simulink model "CAVE_MachE_dSPACE_250912"  (R2024a)
settings: configuration reference "ConfigSetDesktopFixedStep" (kept outside this file)
PreLoadFcn:
  | VSS_BICYCLE=Simulink.Variant('Dual=0');
  | VSS_DUAL=Simulink.Variant('Dual=1');
  | Dual=1;
  | load('DriveCycle2.mat')
PostLoadFcn:
  | if any(exist('dsrtsu_mdlpostloadfcn', 'file') ~= 0), dsrtsu_mdlpostloadfcn('Execute', bdroot); end
InitFcn:
  | , if any(exist('rtifpga_mdlclblib', 'file') ~= 0), rtifpga_mdlclblib('Init', bdroot); end,
  | , if any(exist('dsmpb_private', 'file') ~= 0), dsmpb_private('dsmpb_mdlclblib', 'Init', bdroot); end,
  | load('DriveCycle2.mat')
model workspace (MAT data in the model file):
  Gas = 0.383333333333
values from neighbouring files (symbols this model uses):
  CoastDown =     [Run_Simulink.mat]
  limitedMCT =     [Run_Simulink.mat]
  MCT =     [Run_Simulink.mat]
  pMCT =     [Run_Simulink.mat]
  RealSimPara =     [Run_Simulink.mat]
  Ref_speed = [13 13.007895099 13.015778396 13.023649891 13.031509584 13.039357475 13.047193564 13.055017851 13.062830336 13.070631019 13.0784199 13.086196979 ... (2669 elements, 2669x1)]    [Ref_speed_and_time.mat]
  Ref_time = [0 0.01 0.02 0.03 0.04 0.05 0.06 0.07 0.08 0.09 0.1 0.11 ... (2669 elements, 2669x1)]    [Ref_speed_and_time.mat]
  US06 =     [Run_Simulink.mat]
undefined symbols (not defined in the file or in its folder): AccelCmd, ActTqLF_Nm_, ActTqLR_Nm_, ActTqRF_Nm_, ActTqRR_Nm_, BattChargeLimitMaxPwr, BattChargeLimitSocBpts, BattChargeLimitTbl, BattChrgCapcty, BattDischargeLimitSocBpts, BattDischargeLimitTbl, BattDischargeMaxPwr, BattNumCellsParallel, BattNumCellsSeries, BattOpenVoltCapBpts, BattOpenVoltTbl, BattResistSocBpts, BattResistTbl, BattResistTempBpts, BrakeMaxPrs, BrakeMaxTrq, ChassisDistCg2FrontAxle, ChassisDistCg2RearAxle, ChassisVehMass, CltchCmd, DecelCmd, DiffRatio, DiscIntNeverNeededParam, EnvGravCnst, EnvPrs, EnvTemp, FuelSpecificGrav, GearCmd, h, InitStates, lgSw, MtrEffSpdBpts, MtrEffTbl, MtrEffTrqBpts, MtrPwrMax, MtrTrqMax, SteeringCmd, SupvsryCtrlRegenBrkCutOffTbl, SupvsryCtrlRegenSpdBpts, TestScnrioCycleNum, VEH
libraries: VSIGenLib x122, simulink x112, etargetslib x75, dsmpblib x55, vehdynlibtire x24, CarMaker4SL x20, autolibshared x19, vehdynlibsuspension x14, vehdynlibtirecommon x14, autolibutils x10, VsrLibWheel x8, autolibpowerinfoutils x6
(part 1 of 31)
PreSaveFcn:
  | , if any(exist('dsmpb_private', 'file') ~= 0), dsmpb_private('dsmpb_mdlclblib', 'PreSave', bdroot); end,
CloseFcn:
  | , if any(exist('dsmpb_private', 'file') ~= 0), dsmpb_private('dsmpb_mdlclblib', 'Close', bdroot); end,
settings Model: DataDictionary=DdPassengerEv.sldd  DSMPB_ID_DATA={'18088',struct('BlockId','f88c42c2-e70e-4436-bd85-ff34452e836e','SignalIds',{{'1df572a0-f117-4729-9091-2c1a0a26ec90','0824b86c-995c-4624-95de-4f5a118cf0f7','1af539eb-325a-4e38-9107-84d6b0267392','ebb0fa34-559f-4fe0-b409-8a817ae8753c','d7145080-d35d-4c02-8c9e-cf76ffb14dc2','5075bfde-4142-4aeb-b309-025b37120541','abbab0bd-1456-4252-a37b-ee5f55ea0579','b5d617b8-bb24-4539-9145-e591a0a295f8','7df03788-1936-4801-98c0-dd7f6dfcacba','19949bfb-f246-4995-90e8-29a3751a0fa7','9454b59a-aedd-4270-89a6-1cca43305823','37cf720c-23c2-4b6d-8589-7b035c806643','98db9f76-eafd-4d54-90d2-d997d73b87d4','ff589fc8-5b21-4798-a75e-d26fc35c1fa1','e61b2882-e27e-4f06-b730-5e5281621b34','6605e0e6-8bf3-4a45-a0b0-4b9c1cf463f3','0d0f5161-daad-47a1-bb1d-ec2adbc183ca','48ba6675-0966-4a1c-b127-4f76dca3de94','3c897f11-b2eb-4eb8-b88f-7b7e913c6e41','378f468e-364f-43c5-91f9-fc8ddef6aca6','9c7f20ac-956d-4c19-bdea-31a2a3930ea2','bc252920-9c7c-4b91-a017-ee1d69e3f03c','a5e7a104-8664-4690-a58a-7cbf05737866','fe1cfa34-9b23-4225-85e3-0403f07d36e7','ab40d80a-815e-4994-aacd-e42d283f5b3a','2a4143b2-c438-4d42-997d-0587141eb8f0','2686c37a-8724-40b3-99fb-f8873ba286b8','3707aa1b-88c1-4f14-8f25-f346aa75c252','7413af4b-f834-4020-ad34-3dd98c546e0c','3445835b-9a90-4408-a32d-d76b66b0385b','23c9a144-1259-4fa3-9a16-4a32a7eadff9','5b4206b0-ea89-4111-86f7-7a4fd8c76b72','85c84ea6-72b6-4ccb-9199-727b305580c3','97bb0073-9d03-44a9-972d-49a0eb465678','8c3f0698-b0b6-4624-aa00-3a3096f7cc2f','c968922f-253e-433f-ad46-daf21e902962','21ad150a-19dc-415b-bc1b-b39528ec9221','a3572415-9467-4ff8-a492-c6c1b3cb1b64','700ac678-fb53-40b6-8e97-9eeffe7a1ca8','14ed5f8b-aa1d-402b-b493-5622a729893d','bdbcc0b3-c6a4-485e-8fbf-8c12a8df89e7','7a19cc2b-f06b-466f-ae52-fb8ac6fb0258','87deda6a-2251-4462-8ae0-a20845c776d4','41874d9b-304a-4265-a3a1-69d5c58383ea'}}),'18719',struct('BlockId','79daabbd-4df4-4017-ba65-d977f7e6cd2f','SignalIds',{{'63c99320-3a8a-469e-8a50-5c577229603f'}}),'18720',struct('BlockId','9f21d727-31d5-41b9-aed1-27a40d8edf8b','SignalIds',{{'abab19c9-0d91-46eb-acba-2a4710e305d8','b04a351a-0162-4e76-85ba-be44ac2701ab','ecceff37-eed3-4b02-b10b-52fe944a17cd'}}),'18721',struct('BlockId','5513e588-accc-447f-8233-209349c29c53','SignalIds',{{'cf7c35a9-6bda-4f5f-bfb5-f51ad44c376b'}}),'18722',struct('BlockId','a427ee23-ff95-4a9c-807f-ad2b61c33ee4','SignalIds',{{'b3e368f1-9670-4dd7-aa42-1fcccca64ddf'}}),'18723',struct('BlockId','53805a71-03ad-4b45-a2ab-66e4ec3700d0','SignalIds',{{'0801da20-d997-46db-8512-e37e1180e77c','d193450d-1a5a-4c8d-a2ac-d5fd306fefe3'}}),'18724',struct('BlockId','4d4909f9-4869-4ae2-8541-060fc5e29366','SignalIds',{{'0588d1ac-5d02-4ce0-9f56-5f4e572c1088','c0609b3e-104e-46bb-beb6-dc1d54d218ce','a0011887-c3f0-4769-95be-c916ccb77447','feb7a80d-e7d1-407d-8b44-49f086fb9d8a'}}),'42147',struct('BlockId','7c85148e-c3d7-432d-b81b-e11d436fb266','SignalIds',{{'d5c1f3b5-a22d-40e2-9adf-73dd3a0fe431'}}),'42148',struct('BlockId','5510fdf1-431a-410f-bcea-f7e8f570e2d1','SignalIds',{{'9fce7f97-eda7-4f24-878f-1a643d43b49c'}}),'42149',struct('BlockId','de0e2a2d-bbe1-43d1-85ae-8561a379e07c','SignalIds',{{'e73be657-c71a-4fa8-ab30-d8cdb28be71d'}}),'42224',struct('BlockId','1b1b092f-214b-4a80-b11b-37b75121e53b','SignalIds',{{'856b8b64-1382-4ba0-b818-e91eea7074c9'}}),'42225',struct('BlockId','cfba7721-c5cf-410b-a196-c40269978734','SignalIds',{{'7065876d-b123-4337-8b23-cec9822ec3f7'}}),'42226',struct('BlockId','45b8b98e-f988-42ef-b616-7180bc819cf2','SignalIds',{{'f4c7852e-b78f-4b21-ba9d-e4df57cf05c4'}}),'42232',struct('BlockId','ac7ecc60-8396-40a4-bc17-9f0f3c0759ca','SignalIds',{{'16a26856-ef2a-4966-8200-82aa3fe7ddbf'}}),'42233',struct('BlockId','13dab684-98bf-43e1-8dcd-5e4b904e530a','SignalIds',{{'2a6f66f1-336d-4450-a338-914a295f0636'}}),'42234',struct('BlockId','c2584fdd-8801-464b-b08c-93b745502641','SignalIds',{{'839033fa-96d7-490f-a336-e4074cb0a3a6'}}),'42263',struct('BlockId','5f5bdefb-1809-46da-bb29-06e43cb74cea','SignalIds',{{'9ba80473-de3d-4829-93f9-e3e4218e61ce'}}),'42264',struct('BlockId','3cf8559d-9792-4b7d-b1e9-07d3e8c975ef','SignalIds',{{'f258ffe4-6a36-4981-abe6-f58a11cec6e4'}}),'42772',struct('BlockId','2d079b89-a5d3-43f5-b2da-b67c6c9ddea6','SignalIds',{{'ca22f614-f5f3-4878-a32c-0e537783a285'}}),'42780',struct('BlockId','22a06564-7b80-437f-9a37-5f0480de49c5','SignalIds',{{'d3558271-70a3-4a15-b412-afa96387f019','02a3409b-9f87-437b-bf3a-cc29eabe585b','4dd1ea73-b952-4f27-91e5-448f679ccffd','2dcb7769-2bf3-4424-ac78-eb5f6dd54b66','045c974e-8d31-4d1e-8c69-be2d2594e84a'}}),'42781',struct('BlockId','f3d872af-dc59-442b-a387-2481dd52f459','SignalIds',{{'4ee2bd44-e8da-4e09-8a2d-8bab973be353','ce2328cf-0071-41cb-90b6-53c9d261887b'}}),'42785',struct('BlockId','b01cfdfa-14c4-45c6-876e-4dfb9db42377','SignalIds',{{'34ca8be0-54ab-4d71-8eb9-bde2ffc0f913'}}),'43275',struct('BlockId','53e01b05-b313-4d43-a0e9-b839859eb710','SignalIds',{{'161239c6-78c1-4aea-a8cb-c03beb6ae8ef'}}),'43351',struct('BlockId','937f730a-1a1f-4f40-8fb6-8c70050ca6d4','SignalIds',{{'ee16bc58-de2e-41bd-bfff-f1a6b1cd3b37','b53a6535-30cb-49b2-9826-525fa2ec09db','6c8ffc13-c120-49b6-9460-32fb34ba5a42','39b2e722-7db4-4c66-a473-01b75ecb1f7e','6185bd49-892f-4e96-a0db-104c5534c4be'}}),'49495',struct('BlockId','35ff131a-9de8-4d32-b660-bb6fceef702f','SignalIds',{{'b3d83f02-eed5-45fe-aef0-78174e9f35bd'}}),'49496',struct('BlockId','bf00eff8-ae28-429c-ab8a-46a75e93ba18','SignalIds',{{'86a9df83-1438-4adb-98b7-232805926a36'}}),'49497',struct('BlockId','d54ce848-7528-4eb9-ae42-5423de96ecef','SignalIds',{{'e89a887d-f88e-44f1-b02b-282b9de2f1ab'}}),'49572',struct('BlockId','c08c591c-899c-44b3-88ca-9869f13035b2','SignalIds',{{'eb7d554f-c70c-43ca-87de-5673b1b09813'}}),'49573',struct('BlockId','9ed6cbeb-a118-471e-b0e5-7b29cbd80ac9','SignalIds',{{'e78b4934-46c3-41f5-baf1-b0c8a26c6d3b'}}),'49574',struct('BlockId','61fba3a3-d3ec-4ab0-be81-a8cb14a538ce','SignalIds',{{'aafde299-1c10-4ae2-865d-2eebd2e1d68a'}}),'49580',struct('BlockId','895e4f2c-adf9-4e1f-babd-51f59cfff5b5','SignalIds',{{'825a4d44-3ac8-4ffd-9f33-50dd2ede91f2'}}),'49581',struct('BlockId','65ead0f7-0652-4680-9e89-6e39b662d157','SignalIds',{{'833f3807-08e2-419e-8eac-d416545ff0e8'}}),'49582',struct('BlockId','ae266637-3823-4e51-9a5d-b81a88878ea4','SignalIds',{{'7abd4bb8-4f81-4261-991b-ba40c4239b3f'}}),'49611',struct('BlockId','77863ddb-e348-485a-81f5-f37c73594fca','SignalIds',{{'b85974cd-0117-43cc-9e24-4cf6f83a5038'}}),'49612',struct('BlockId','8a6bfe7e-fecd-4338-b064-35f762c57dd4','SignalIds',{{'028a9207-fccc-429b-a69c-4f023900ccb5'}}),'50148',struct('BlockId','d1cbcaa1-cb10-47dc-bb74-55eff0f5b43b','SignalIds',{{'203ceee9-7451-4837-a304-33672f7cb3bd'}}),'50156',struct('BlockId','7627d88c-f2e4-403d-80ba-43b5276eda68','SignalIds',{{'322b732d-d2d2-46e4-9338-f008ec14fc06','19c378a0-40df-4104-b400-16195277658b','129b4dde-e693-4553-ada1-0a9cf8694d1d','28bef0ec-e017-4484-a602-27bf02ddcdfb','d37ce16d-143d-4750-b239-1ca329bec6cc'}}),'50157',struct('BlockId','caace046-61cc-4e48-8b3d-a44e7bf76e0c','SignalIds',{{'2a1998fe-82ad-4e18-9452-adc54fc26a08','16216acf-8215-436c-93b3-ee24dac643a7'}}),'50161',struct('BlockId','87d87a7c-a686-43fe-9c61-68513704cc99','SignalIds',{{'b845dc9e-5d72-4a9d-93ac-413a3cfc992f'}}),'50651',struct('BlockId','00e0e527-d2ca-4571-801c-cfc2bc29d995','SignalIds',{{'b4404b90-9372-444b-968a-2bd31005b611'}}),'50727',struct('BlockId','25b59a2e-42b7-4e07-879c-15e188342b70','SignalIds',{{'e976513c-fd89-4869-a98f-324219a9d934','829bf17c-2f45-4024-9dab-76a03bee14cf','0e1b211c-e5c6-4562-ba57-cff21183358a','56f35125-16f5-4225-9f4e-e6e61c42686e','40167815-fad9-4050-b1e6-1da6841d0f65'}}),'53300',struct('BlockId','ae15802c-8b47-4761-960d-0ebe7bc28239','SignalIds',{{'650e13a2-8980-4a2b-ad4a-82bd33536a23'}}),'53322',struct('BlockId','ff36f65e-48c3-4e0a-8bc0-4b163bd9adbf','SignalIds',{{'5a20c0d4-68ad-414c-b231-cbf9ddd3e095'}}),'53323',struct('BlockId','ff546a49-594f-4f8a-affd-90d138806f61','SignalIds',{{'5fe60c73-3931-4298-88e1-7e5400488d1f','248c84a0-5741-40b6-9df8-c31abbb2257e','cca71626-162d-41c0-b616-b3a204f50bd7','6e7b0574-cba0-4ecc-ac4f-9c1d2acf4299'}}),'53324',struct('BlockId','a705fb28-535c-4f81-ad43-e460cea2d9bd','SignalIds',{{'398a40fd-c49e-4cdc-b573-2bb4186f6a80'}}),'53325',struct('BlockId','640f6546-7547-4622-bc5f-0a859f60736c','SignalIds',{{'f16056a3-5355-45cf-b9ed-57b3d5aab693'}}),'53330',struct('BlockId','93c276bb-de34-4a5c-95b3-f478e766cc9c','SignalIds',{{'c132201b-d036-47bb-91a2-a150e3b7ae13','ab601218-fa7c-4092-949e-1c1efb88023c'}}),'53343',struct('BlockId','8d0d14d0-22eb-49b1-810b-505b992714e9','SignalIds',{{'23156721-17dc-438a-8419-66eeaab95ef6','031c7289-7cec-4992-a9bf-cac5b5fae03e','ee32aa15-99a4-47b6-971a-419c12efa46a'}}),'53436',struct('BlockId','f41b78f3-d575-41ef-a146-3918605c1ef5','SignalIds',{{'e2c9672b-95ca-4046-bb0a-7aa2ea23f667'}}),'53439',struct('BlockId','d56f2d58-e632-40cf-b303-c9d86bf84e1a','SignalIds',{{'59ee7074-abb0-4813-a7c7-2ef1cc941406'}}),'53488',struct('BlockId','418072fe-6709-46db-9629-338ace776db3','SignalIds',{{'044486e3-c8e5-469a-9e14-4b7ebf45cbba','40dd4e22-2973-48dc-8d39-42c08d6738c4'}}),'53490',struct('BlockId','7526ad31-4259-4e92-8867-16b3b004889f','SignalIds',{{'fba7c128-fffd-4ae7-8d8c-de066c2017dd'}}),'53491',struct('BlockId','062ca957-a507-4bdc-8288-474fbe5dbd0f','SignalIds',{{'af7253ef-dad5-44d9-bc07-eac7de166a86','3be6fa1b-709c-42ac-b822-ca052c4e2367','f965bb3f-6162-4a13-806f-161423ed84b7'}}),'53492',struct('BlockId','fc9bee8e-3606-4482-8e61-57f769d8705e','SignalIds',{{'08427df5-b687-45d9-8b32-97283f4d5ce7'}}),'53509',struct('BlockId','bc68f02f-4d7c-4dde-a2d1-5019dce219ff','SignalIds',{{'21518aaf-593c-482f-a05c-e4a1b5e97c9f','b433a259-e771-4f81-a0d0-6fb158bd2e5d','6775e424-27e2-42c2-9fab-4841f171aca3','bf8792cd-664c-41ca-8c7b-827f476f84f2'}})}  RTICANMMDATA=struct('GeneralSetupData',struct('modelroot','C:\GitDev\Anye\cave_carla_dev\Vehicles\VehicleProjects\Bolt_EV\System','generalsettings',struct('filesettings',struct('destfolder',struct('Name','RTICANMM_FILES','Check',1),'buildfolder',struct('Name','.','Check',1),'AbsDestfolder',struct('Name','C:\GitDev\Anye\cave_carla_dev\Vehicles\VehicleProjects\Bolt_EV\System\RTICANMM_FILES'),'AbsBuildfolder',struct('Name','C:\GitDev\Anye\cave_carla_dev\Vehicles\VehicleProjects\Bolt_EV\System'))),'options',struct('addpaths',1,'rmpaths',1,'addtrcexclusion',true,'cannavigator',struct('checkmonitoring',0),'show_usrtrc',0,'use_usrtrc',0),'advanced',struct('options',ones(1,100)),'MPSetup',{{}},'RTI',struct('Type','DSRT','Ver','4.2p1','Date','11-Feb-2020'),'modelname','CAVE_MachE','block','CAVE_MachE'))  DSRTSU_INTERNAL_RTIFPGA=210  DSRTSU_INTERNAL_RTISTBM_VER=24.1  PauseTimes=45  Creator=9bt  LastModifiedBy=MSC_Lab
settings ConfigSetRef: SourceName=ConfigSetDesktopFixedStep

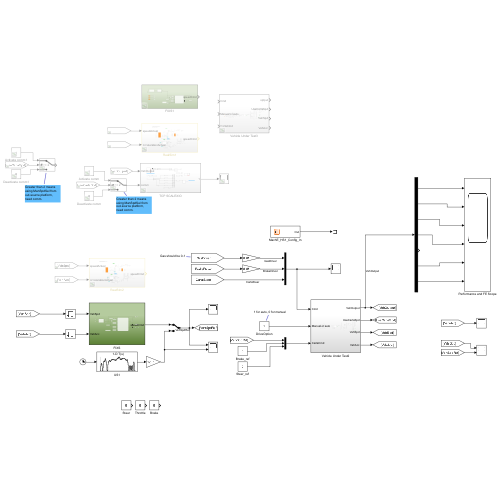
[thumbnail: Simulink's stored preview of the top-level diagram]
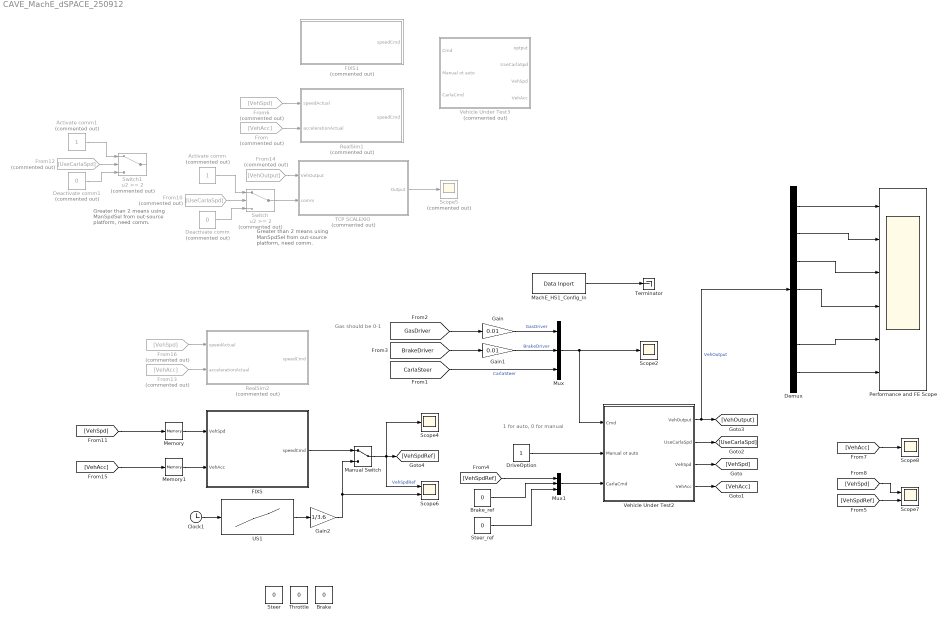
== system CAVE_MachE_dSPACE_250912 ==
  note: Greater than 2 means using ManSpdSel from out-source platform, need comm.
  note: 1 for auto, 0 for manual
  note: Gas should be 0-1
  note: Greater than 2 means using ManSpdSel from out-source platform, need comm.
  Activate comm : Constant  Commented=on
  Activate comm1 : Constant  Commented=on
  Brake : Constant  Value=0
  Brake_ref : Constant  Value=0
  Clock1 : Clock
  Deactivate comm : Constant  Commented=on  Value=0
  Deactivate comm1 : Constant  Commented=on  Value=0
  Demux : Demux  Outputs=7
  DriveOption : Constant
  FIXS : Subsystem
  FIXS1 : Subsystem  Commented=on
  From : From  Commented=on  GotoTag=VehAcc
  From10 : From  Commented=on  GotoTag=UseCarlaSpd
  From12 : From  Commented=on  GotoTag=UseCarlaSpd
  From13 : From  Commented=on  GotoTag=VehAcc
  From14 : From  Commented=on  GotoTag=VehOutput
  From16 : From  Commented=on  GotoTag=VehSpd
  From6 : From  Commented=on  GotoTag=VehSpd
  Gain : Gain  Gain=0.01
  Gain1 : Gain  Gain=0.01
  Gain2 : Gain  Gain=1/3.6
  MachE_HS1_Config_In : dsmpblib/Data Inport  Priority=10000
      settings: SourceProductName=dSPACE Model Interface Package for Simulink (MIPS)
  Manual Switch : ManualSwitch
  Memory : Memory
  Memory1 : Memory
  Mux : Mux  Inputs=3
  Mux1 : Mux  Inputs=3
  Performance and FE Scope : Scope  NumInputPorts=6
  RealSim1 : Subsystem  Commented=on
  RealSim2 : Subsystem  Commented=on
  Scope2 : Scope
  Scope4 : Scope
  Scope5 : Scope  Commented=on
  Scope6 : Scope  NumInputPorts=2
  Scope7 : Scope  NumInputPorts=2
  Scope8 : Scope
  Steer : Constant  Value=0
  Steer_ref : Constant  Value=0
  Switch : Switch  Commented=on  Threshold=2  SaturateOnIntegerOverflow=off  InputSameDT=off
  Switch1 : Switch  Commented=on  Threshold=2  SaturateOnIntegerOverflow=off  InputSameDT=off
  TCP SCALEXIO : Subsystem  Commented=on
  Terminator : Terminator
  Throttle : Constant  Value=0
  US1 : Lookup_n-D  NumberOfTableDimensions=1  BreakpointsForDimension1=US06.Time  Table=US06.Speed  InternalRulePriority=Speed  RndMeth=Simplest
  Vehicle Under Test2 : Subsystem
  Vehicle Under Test3 : Subsystem  Commented=on
  wires:
  Mux/1 -> Vehicle Under Test2/1(Cmd), Scope2/1
  DriveOption/1 -> Vehicle Under Test2/2(Manual ot auto)
  [GasDriver] -> Gain/1
  [BrakeDriver] -> Gain1/1
  MachE_HS1_Config_In/1 -> Terminator/1
  Gain/1 -> Mux/1  "GasDriver"
  Gain1/1 -> Mux/2  "BrakeDriver"
  Vehicle Under Test2/1(VehOutput) -> [VehOutput], Demux/1  "VehOutput"
  Switch/1 -> TCP SCALEXIO/2(comm)
  TCP SCALEXIO/1(Output) -> Scope5/1
  Deactivate comm/1 -> Switch/3
  Activate comm/1 -> Switch/1
  [CarlaSteer] -> Mux/3  "CarlaSteer"
  Manual Switch/1 -> Scope4/1, Scope6/1, [VehSpdRef]  "VehSpdRef"
  US1/1 -> Gain2/1
  From/1 -> RealSim1/2(accelerationActual)
  From6/1 -> RealSim1/1(speedActual)
  [VehSpdRef] -> Mux1/1
  Mux1/1 -> Vehicle Under Test2/3(CarlaCmd)
  Vehicle Under Test2/3(VehSpd) -> [VehSpd]
  Vehicle Under Test2/4(VehAcc) -> [VehAcc]
  Steer_ref/1 -> Mux1/3
  Brake_ref/1 -> Mux1/2
  Vehicle Under Test2/2(UseCarlaSpd) -> [UseCarlaSpd]
  Clock1/1 -> US1/1
  [VehSpdRef] -> Scope7/2
  Gain2/1 -> Scope6/2, Manual Switch/2
  Demux/1 -> Performance and FE Scope/1
  Demux/7 -> Performance and FE Scope/6
  Demux/6 -> Performance and FE Scope/5
  Demux/4 -> Performance and FE Scope/4
  Demux/3 -> Performance and FE Scope/3
  Demux/2 -> Performance and FE Scope/2
  [VehAcc] -> Scope8/1
  [VehSpd] -> Scope7/1
  From10/1 -> Switch/2
  [VehSpd] -> Memory/1
  FIXS/1(speedCmd) -> Manual Switch/1
  From12/1 -> Switch1/2
  Activate comm1/1 -> Switch1/1
  Deactivate comm1/1 -> Switch1/3
  From14/1 -> TCP SCALEXIO/1(VehOutput)
  [VehAcc] -> Memory1/1
  From16/1 -> RealSim2/1(speedActual)
  From13/1 -> RealSim2/2(accelerationActual)
  Memory/1 -> FIXS/1(VehSpd)
  Memory1/1 -> FIXS/2(VehAcc)

== system CAVE_MachE_dSPACE_250912/FIXS ==
  note: This flag will bypass all other logic and force the ramp down of HIL
  VehSpd : Inport
  VehAcc : Inport  Port=2
  Clock : Clock
  Constant : Constant  Value=RealSimPara.speedInit
  DistanceTravel (m) : Constant  Value=0
  Gain3 : Gain  Gain=3.6
  Manual Switch : ManualSwitch  CurrentSetting=0
  Manual Switch1 : ManualSwitch
  RampDownFlag : Constant  Value=0
  RampUpFlag : Constant  Value=0
  RealSim Core : Subsystem
  RealSimHILCycle : Stateflow chart  TreatAsAtomicUnit=on
  SimState : Constant  Value=10
  SimTime : Constant  Value=10
  Terminator{,1..4} (5 alike) : Terminator
  initialWaitTime : Constant  Value=0
  totalDistance (m) : Constant  Value=1000000
  totalTime (sec) : Constant  Value=10000
  speedCmd : Outport
  wires:
  RealSim Core/2(speedDesiredIn) -> Terminator/1
  RampDownFlag/1 -> RealSimHILCycle/9(RampDownFlag)
  totalDistance (m)/1 -> RealSimHILCycle/7(totalDistance)
  Manual Switch/1 -> RealSimHILCycle/3(SpeedIn)
  Gain3/1 -> Terminator1/1  "HIL_SpeedCmd_kph"
  totalTime (sec)/1 -> RealSimHILCycle/8(totalTime)
  RealSimHILCycle/1(CycleMode) -> Terminator3/1  "CycleMode"
  initialWaitTime/1 -> RealSimHILCycle/5(InitWaitTime)
  RealSimHILCycle/2(SpeedCmd) -> [HIL_SpeedCmd], Manual Switch1/2, Gain3/1
  Constant/1 -> Manual Switch/1, RealSimHILCycle/6(SpeedInit)
  Manual Switch1/1 -> speedCmd/1
  RealSim Core/3(speedCmd) -> Manual Switch1/1, Manual Switch/2
  RampUpFlag/1 -> RealSimHILCycle/10(RampUpFlag)
  VehSpd/1 -> RealSim Core/1(VehSpd)
  RealSim Core/1(VehDataBusIn) -> Terminator2/1
  RealSim Core/4(speedActual) -> Terminator4/1
  DistanceTravel (m)/1 -> RealSimHILCycle/4(DistanceTravel)
  SimState/1 -> RealSimHILCycle/2(SimState)
  Clock/1 -> RealSimHILCycle/1(SimTime)
  VehAcc/1 -> RealSim Core/2(VehAcc)

== system CAVE_MachE_dSPACE_250912/FIXS1 ==
  note: This flag will bypass all other logic and force the ramp down of HIL
  Constant : Constant  Value=RealSimPara.speedInit
  Gain3 : Gain  Gain=3.6
  Manual Switch : ManualSwitch  CurrentSetting=0
  Manual Switch1 : ManualSwitch  CurrentSetting=0
  RampDownFlag : Constant  Value=0
  RampUpFlag : Constant  Value=0
  Read CM Dict3 : CarMaker4SL/Read CM Dict  xname=Time  xsync=off  xstime=Continuous
  Read CM Dict7 : CarMaker4SL/Read CM Dict  xname=SC.State  xsync=off  xstime=Continuous
  Read CM Dict8 : CarMaker4SL/Read CM Dict  xname=Vhcl.Distance  xsync=off  xstime=Continuous
  RealSim Core : Subsystem
  RealSim Translate CM Signal to Bus as Feedback to SUMO/VISSIM : Subsystem
  RealSimHILCycle : Stateflow chart  TreatAsAtomicUnit=on
  Terminator : Terminator
  Terminator1 : Terminator
  Terminator3 : Terminator
  initialWaitTime : Constant  Value=10000
  totalDistance (m) : Constant  Value=1000000
  totalTime (sec) : Constant  Value=10000
  speedCmd : Outport
  wires:
  RealSim Translate CM Signal to Bus as Feedback to SUMO/VISSIM/1(VehDataBusOut) -> RealSim Core/1(VehDataBusOut)
  RealSim Core/2(speedDesiredIn) -> Terminator/1
  RealSim Core/1(VehDataBusIn) -> RealSim Translate CM Signal to Bus as Feedback to SUMO/VISSIM/1(VehDataBusIn)
  RealSim Translate CM Signal to Bus as Feedback to SUMO/VISSIM/2(CM_speed) -> RealSim Core/2(CM_speed)
  RampDownFlag/1 -> RealSimHILCycle/9(RampDownFlag)
  totalDistance (m)/1 -> RealSimHILCycle/7(totalDistance)
  Manual Switch/1 -> RealSimHILCycle/3(SpeedIn)
  Gain3/1 -> Terminator1/1  "HIL_SpeedCmd_kph"
  totalTime (sec)/1 -> RealSimHILCycle/8(totalTime)
  RealSimHILCycle/1(CycleMode) -> Terminator3/1  "CycleMode"
  initialWaitTime/1 -> RealSimHILCycle/5(InitWaitTime)
  RealSimHILCycle/2(SpeedCmd) -> [HIL_SpeedCmd], Manual Switch1/2, Gain3/1
  Constant/1 -> RealSimHILCycle/6(SpeedInit), Manual Switch/1
  [DistanceTravel] -> RealSimHILCycle/4(DistanceTravel)
  [SimState] -> RealSimHILCycle/2(SimState)
  [CM_Time] -> RealSimHILCycle/1(SimTime)
  Manual Switch1/1 -> speedCmd/1
  RealSim Core/3(speedCmd) -> Manual Switch/2, Manual Switch1/1
  Read CM Dict7/1 -> [SimState]  "SimCore_State"
  Read CM Dict8/1 -> [DistanceTravel]  "distanceTravel"
  Read CM Dict3/1 -> [CM_Time]  "CM_Time"
  RampUpFlag/1 -> RealSimHILCycle/10(RampUpFlag)
  RealSim Core/4(speedActual) -> RealSim Translate CM Signal to Bus as Feedback to SUMO/VISSIM/2(speedActual)

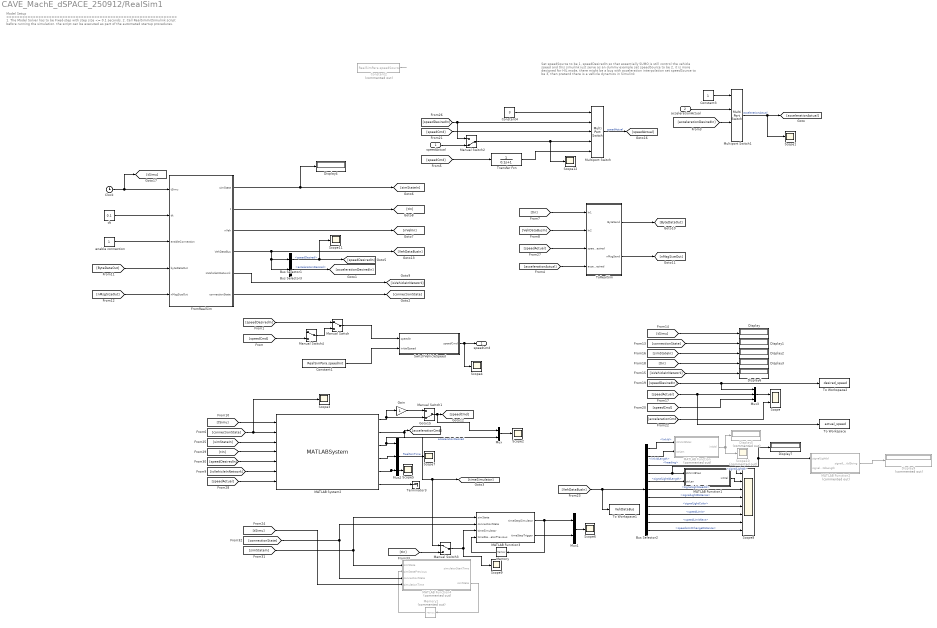
== system CAVE_MachE_dSPACE_250912/RealSim1 ==
  note: Set speedSource to be 1, speedDesiredIn so that essentially SUMO is still control the vehicle speed and this simulink just serve as an dummy example
      |
      | set speedSource to be 2, it is more designed for HIL mode, there might be a bug with acceleration interpolation
      |
      | set speedSource to be 3, then pretend there is a vehicle dynamics in Simulink
  note: Model Setup
      | ================================================================
      | 1. The Model Solver has to be Fixed-step with step size <= 0.1 seconds.
      | 2. Call RealSimInitSimulink script before running the simulation. the script can be executed as part of the automated startup procedures.
  speedActual : Inport
  accelerationActual : Inport  Port=2
  Bus Selector1 : BusSelector  OutputSignals=speedDesired
  Bus Selector2 : BusSelector  OutputSignals=linkId,linkIdLength,heading,signalLightId,signalLightIdLength,signalLightHeadId,signalLightDistance,signalLightColor,speedLimit,speedLimitNext,speedLimitChangeDistance
  Bus Selector3 : BusSelector  OutputSignals=accelerationDesired
  Clock : Clock
  Constant1 : Constant  Value=RealSimPara.speedInit
  Constant2 : Constant  Commented=on  Value=RealSimPara.speedSource
  Constant3 : Constant
  Constant4 : Constant  Value=3
  Display{,1..4,6..7} (7 alike) : Display
  Display5 : Display  Commented=on
  Display9 : Display  Commented=on
  FromRealSim : Subsystem
  Gain : Gain
  MATLAB Function : MATLAB Function  Commented=on  TreatAsAtomicUnit=on
  MATLAB Function1 : MATLAB Function  TreatAsAtomicUnit=on
  MATLAB Function2 : MATLAB Function  Commented=on  TreatAsAtomicUnit=on  SystemSampleTime=0.001
  MATLAB Function3 : MATLAB Function  TreatAsAtomicUnit=on
  MATLAB Function4 : MATLAB Function  Commented=on  TreatAsAtomicUnit=on
  MATLAB System2 : MATLABSystem  System=RealSimInterpSpeed  initialSpeed=RealSimPara.speedInit  speedLookAheadHorizon=RealSimPara.tLookahead  speedUpperBound=30  smoothWindow=RealSimPara.smoothWindow  SimulateUsing=Interpreted execution
      mask Type: RealSimInterpSpeed
      mask Display:
      | disp('RealSimInterpSpeed');
      | port_label('input',1,'simulationTime');
      | port_label('input',2,'connectionState');
      | port_label('input',3,'simState');
      | port_label('input',4,'timeReceive');
      | port_label('input',5,'speedReceive');
      | port_label('input',6,'isVehicleInNetwork');
      | port_label('input',7,'speedActual');
      | port_label('output',1,'speedLookAhead');
      | port_label('output',2,'accelerationDesired');
      | port_label('output',3,'timeSimulator');
      | port_label('output',4,'timeStepSimulator');
      | port_label('output',5,'timeStepTrigger');
      | port_label('output',6,'RealSimDelay');
  Manual Switch : ManualSwitch
  Manual Switch1 : ManualSwitch  CurrentSetting=0
  Manual Switch2 : ManualSwitch  CurrentSetting=0
  Manual Switch3 : ManualSwitch
  Manual Switch4 : ManualSwitch
  Memory : Memory
  Memory1 : Memory  Commented=on
  Multiport Switch : MultiPortSwitch  Inputs=4  SaturateOnIntegerOverflow=off  InputSameDT=off
  Multiport Switch1 : MultiPortSwitch  SaturateOnIntegerOverflow=off  InputSameDT=off
  Mux : Mux  Inputs=2
  Mux1 : Mux  Inputs=2
  Mux2 : Mux  Inputs=3
  Mux3 : Mux  Inputs=3
  Scope : Scope  NumInputPorts=2
  Scope{1..7,9,11..12} (10 alike) : Scope
  Scope10 : Scope  Commented=on
  Scope8 : Scope  NumInputPorts=8
  SwitchVehicleSpeed : Subsystem
  Terminator3 : Terminator
  To Workspace : ToWorkspace  VariableName=actual_speed  SaveFormat=Timeseries  SampleTime=0.1
  To Workspace1 : ToWorkspace  VariableName=VehDataBus  SaveFormat=Timeseries  SampleTime=-1
  To Workspace2 : ToWorkspace  VariableName=desired_speed  SaveFormat=Timeseries  SampleTime=0.1
  ToRealSim : Subsystem
  Transfer Fcn : TransferFcn  Denominator=[0.1 1]
  dt : Constant  Value=0.1
  enable connection : Constant
  speedCmd : Outport
  wires:
  [speedCmd] -> Manual Switch4/2
  Manual Switch3/1 -> MATLAB Function3/3(timeSimulator), Scope9/1
  [tIn] -> Manual Switch3/2
  MATLAB Function4/2(simState) -> Memory1/1
  Memory1/1 -> MATLAB Function4/2(simStatePrevious)
  MATLAB Function3/2(timeStepTrigger) -> Mux1/2
  Mux1/1 -> Scope6/1
  Memory/1 -> MATLAB Function3/4(timeStepSimulatorPrevious)
  MATLAB Function3/1(timeStepSimulator) -> Memory/1, Mux1/1
  [simStateIn] -> MATLAB Function3/1(simState), MATLAB Function4/1("simState ")
  [connectionState] -> MATLAB Function3/2(connectionState), MATLAB Function4/3(connectionState)
  [tSimu] -> MATLAB Function4/4(simulationTime)
  Transfer Fcn/1 -> Multiport Switch/5
  [speedCmd] -> Transfer Fcn/1
  speedActual/1 -> Manual Switch2/2
  Mux/1 -> Scope2/1
  FromRealSim/6(connectionState) -> [connectionState]
  Multiport Switch1/1 -> [accelerationActual], Scope1/1  "accelerationActual"
  accelerationActual/1 -> Multiport Switch1/2
  [accelerationDesiredIn] -> Multiport Switch1/3
  Constant3/1 -> Multiport Switch1/1
  Bus Selector3/1 -> [accelerationDesiredIn]  "<accelerationDesired>"
  Manual Switch/1 -> SwitchVehicleSpeed/1(speedIn)
  SwitchVehicleSpeed/1(speedCmd) -> speedCmd/1, Scope4/1
  Constant1/1 -> SwitchVehicleSpeed/2(initialSpeed)
  [speedDesiredIn] -> Manual Switch/1
  Manual Switch4/1 -> Manual Switch/2
  Constant2/1 -> ?
  ? -> MATLAB Function2/2(signalLightIdLength)
  [simStateIn] -> Display2/1
  Mux3/1 -> Scope/1
  [isVehicleInNetwork] -> MATLAB System2/6
  Bus Selector2/3 -> Scope8/1  "<heading>"
  MATLAB Function1/1(intVal) -> Scope8/2
  ToRealSim/1(ByteSend) -> [ByteDataOut]
  [accelerationActual] -> ToRealSim/4(accelerationDesired)
  Bus Selector2/6 -> Scope8/3  "<signalLightHeadId>"
  Multiport Switch/1 -> [speedActual]  "speedActual"
  [VehDataBusIn] -> ToRealSim/2(In2)
  [accelerationCmd] -> Scope/2
  FromRealSim/5(isVehicleInNetwork) -> [isVehicleInNetwork]
  FromRealSim/2(t) -> [tIn]
  [speedActual] -> ToRealSim/3(speedDesired)
  FromRealSim/1(simState) -> [simStateIn], Display4/1
  ToRealSim/2(nMsgSend) -> [nMsgSizeOut]
  Manual Switch1/1 -> [speedCmd], Mux/1
  Constant4/1 -> Multiport Switch/1
  [speedCmd] -> Mux3/3
  [tIn] -> MATLAB System2/4
  Bus Selector2/2 -> MATLAB Function/2(strLen)  "<linkIdLength>"
  MATLAB Function2/1(signalLightIdString) -> Display9/1
  MATLAB System2/2 -> Mux/2, [accelerationCmd]  "accelerationDesired"
  [tIn] -> ToRealSim/1(In1)
  Bus Selector2/1 -> MATLAB Function/1(strUint8Vec)  "<linkId>"
  MATLAB System2/6 -> Terminator3/1
  [connectionState] -> Scope3/1, MATLAB System2/2
  Manual Switch2/1 -> Multiport Switch/4, Scope12/1
  Bus Selector2/8 -> Scope8/5  "<signalLightColor>"
  MATLAB System2/4 -> Mux2/2
  Bus Selector2/7 -> Scope8/4  "<signalLightDistance>"
  [tIn] -> Display3/1
  Clock/1 -> [tSimu], FromRealSim/1(tSimu)
  [connectionState] -> Display1/1
  [speedActual] -> Mux3/2, To Workspace/1
  FromRealSim/3(nVeh) -> [nVehIn]
  [speedActual] -> MATLAB System2/7
  [speedDesiredIn] -> Multiport Switch/2, Manual Switch2/1
  Bus Selector2/11 -> Scope8/8  "<speedLimitChangeDistance>"
  [nMsgSizeOut] -> FromRealSim/5(nMsgSizeOut)
  [speedDesiredIn] -> MATLAB System2/5
  MATLAB Function/1(intVal) -> Display5/1, Scope10/1
  enable connection/1 -> FromRealSim/3(enableConnection)
  FromRealSim/4(VehDataBus) -> Bus Selector3/1, Bus Selector1/1, [VehDataBusIn]
  Bus Selector2/10 -> Scope8/7  "<speedLimitNext>"
  dt/1 -> FromRealSim/2(dt)
  MATLAB System2/3 -> Mux2/1, Manual Switch3/1, [timeSimulator]
  Bus Selector2/4 -> MATLAB Function1/1(strUint8Vec), MATLAB Function2/1(signalLightId), Display7/1  "<signalLightId>"
  [speedDesiredIn] -> Mux3/1, To Workspace2/1
  Bus Selector2/9 -> Scope8/6  "<speedLimit>"
  Bus Selector1/1 -> [speedDesiredIn], Scope11/1  "<speedDesired>"
  Gain/1 -> Manual Switch1/1
  [tSimu] -> MATLAB System2/1
  Mux2/1 -> Scope7/1  "RealSimTime"
  [speedCmd] -> Multiport Switch/3
  MATLAB System2/1 -> Manual Switch1/2, Gain/1
  [VehDataBusIn] -> Bus Selector2/1, To Workspace1/1
  MATLAB System2/5 -> Mux2/3, Scope5/1
  [ByteDataOut] -> FromRealSim/4(byteDataOut)
  [isVehicleInNetwork] -> Display6/1
  [simStateIn] -> MATLAB System2/3
  Bus Selector2/5 -> MATLAB Function1/2(strLen)  "<signalLightIdLength>"
  [tSimu] -> Display/1

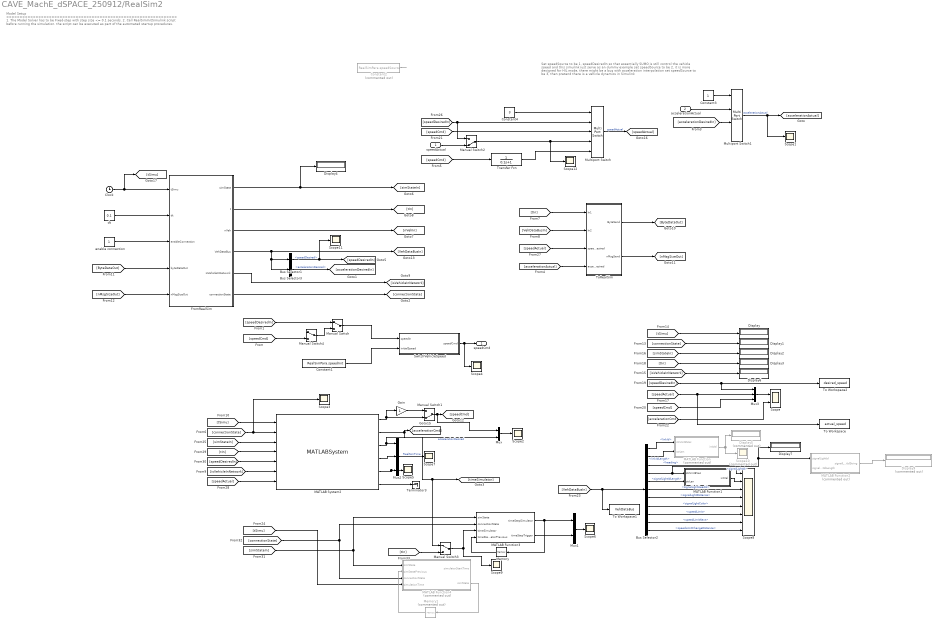
== system CAVE_MachE_dSPACE_250912/RealSim2 ==
  note: Model Setup
      | ================================================================
      | 1. The Model Solver has to be Fixed-step with step size <= 0.1 seconds.
      | 2. Call RealSimInitSimulink script before running the simulation. the script can be executed as part of the automated startup procedures.
  note: Set speedSource to be 1, speedDesiredIn so that essentially SUMO is still control the vehicle speed and this simulink just serve as an dummy example
      |
      | set speedSource to be 2, it is more designed for HIL mode, there might be a bug with acceleration interpolation
      |
      | set speedSource to be 3, then pretend there is a vehicle dynamics in Simulink
  speedActual : Inport
  accelerationActual : Inport  Port=2
  Bus Selector1 : BusSelector  OutputSignals=speedDesired
  Bus Selector2 : BusSelector  OutputSignals=linkId,linkIdLength,heading,signalLightId,signalLightIdLength,signalLightHeadId,signalLightDistance,signalLightColor,speedLimit,speedLimitNext,speedLimitChangeDistance
  Bus Selector3 : BusSelector  OutputSignals=accelerationDesired
  Clock : Clock
  Constant1 : Constant  Value=RealSimPara.speedInit
  Constant2 : Constant  Commented=on  Value=RealSimPara.speedSource
  Constant3 : Constant
  Constant4 : Constant  Value=3
  Display{,1..4,6..7} (7 alike) : Display
  Display5 : Display  Commented=on
  Display9 : Display  Commented=on
  FromRealSim : Subsystem
  Gain : Gain
  MATLAB Function : MATLAB Function  Commented=on  TreatAsAtomicUnit=on
  MATLAB Function1 : MATLAB Function  TreatAsAtomicUnit=on
  MATLAB Function2 : MATLAB Function  Commented=on  TreatAsAtomicUnit=on  SystemSampleTime=0.001
  MATLAB Function3 : MATLAB Function  TreatAsAtomicUnit=on
  MATLAB Function4 : MATLAB Function  Commented=on  TreatAsAtomicUnit=on
  MATLAB System2 : MATLABSystem  System=RealSimInterpSpeed  initialSpeed=RealSimPara.speedInit  speedLookAheadHorizon=RealSimPara.tLookahead  speedUpperBound=30  smoothWindow=RealSimPara.smoothWindow  SimulateUsing=Interpreted execution
      mask Type: RealSimInterpSpeed
      mask Display:
      | disp('RealSimInterpSpeed');
      | port_label('input',1,'simulationTime');
      | port_label('input',2,'connectionState');
      | port_label('input',3,'simState');
      | port_label('input',4,'timeReceive');
      | port_label('input',5,'speedReceive');
      | port_label('input',6,'isVehicleInNetwork');
      | port_label('input',7,'speedActual');
      | port_label('output',1,'speedLookAhead');
      | port_label('output',2,'accelerationDesired');
      | port_label('output',3,'timeSimulator');
      | port_label('output',4,'timeStepSimulator');
      | port_label('output',5,'timeStepTrigger');
      | port_label('output',6,'RealSimDelay');
  Manual Switch : ManualSwitch
  Manual Switch1 : ManualSwitch  CurrentSetting=0
  Manual Switch2 : ManualSwitch  CurrentSetting=0
  Manual Switch3 : ManualSwitch
  Manual Switch4 : ManualSwitch
  Memory : Memory
  Memory1 : Memory  Commented=on
  Multiport Switch : MultiPortSwitch  Inputs=4  SaturateOnIntegerOverflow=off  InputSameDT=off
  Multiport Switch1 : MultiPortSwitch  SaturateOnIntegerOverflow=off  InputSameDT=off
  Mux : Mux  Inputs=2
  Mux1 : Mux  Inputs=2
  Mux2 : Mux  Inputs=3
  Mux3 : Mux  Inputs=3
  Scope : Scope  NumInputPorts=2
  Scope{1..7,9,11..12} (10 alike) : Scope
  Scope10 : Scope  Commented=on
  Scope8 : Scope  NumInputPorts=8
  SwitchVehicleSpeed : Subsystem
  Terminator3 : Terminator
  To Workspace : ToWorkspace  VariableName=actual_speed  SaveFormat=Timeseries  SampleTime=0.1
  To Workspace1 : ToWorkspace  VariableName=VehDataBus  SaveFormat=Timeseries  SampleTime=-1
  To Workspace2 : ToWorkspace  VariableName=desired_speed  SaveFormat=Timeseries  SampleTime=0.1
  ToRealSim : Subsystem
  Transfer Fcn : TransferFcn  Denominator=[0.1 1]
  dt : Constant  Value=0.1
  enable connection : Constant
  speedCmd : Outport
  wires:
  [tSimu] -> Display/1
  Bus Selector2/5 -> MATLAB Function1/2(strLen)  "<signalLightIdLength>"
  [simStateIn] -> MATLAB System2/3
  [isVehicleInNetwork] -> Display6/1
  [ByteDataOut] -> FromRealSim/4(byteDataOut)
  MATLAB System2/5 -> Scope5/1, Mux2/3
  [VehDataBusIn] -> To Workspace1/1, Bus Selector2/1
  MATLAB System2/1 -> Gain/1, Manual Switch1/2
  [speedCmd] -> Multiport Switch/3
  Mux2/1 -> Scope7/1  "RealSimTime"
  [tSimu] -> MATLAB System2/1
  Gain/1 -> Manual Switch1/1
  Bus Selector1/1 -> Scope11/1, [speedDesiredIn]  "<speedDesired>"
  Bus Selector2/9 -> Scope8/6  "<speedLimit>"
  [speedDesiredIn] -> To Workspace2/1, Mux3/1
  Bus Selector2/4 -> Display7/1, MATLAB Function2/1(signalLightId), MATLAB Function1/1(strUint8Vec)  "<signalLightId>"
  MATLAB System2/3 -> [timeSimulator], Manual Switch3/1, Mux2/1
  dt/1 -> FromRealSim/2(dt)
  Bus Selector2/10 -> Scope8/7  "<speedLimitNext>"
  FromRealSim/4(VehDataBus) -> [VehDataBusIn], Bus Selector1/1, Bus Selector3/1
  enable connection/1 -> FromRealSim/3(enableConnection)
  MATLAB Function/1(intVal) -> Scope10/1, Display5/1
  [speedDesiredIn] -> MATLAB System2/5
  [nMsgSizeOut] -> FromRealSim/5(nMsgSizeOut)
  Bus Selector2/11 -> Scope8/8  "<speedLimitChangeDistance>"
  [speedDesiredIn] -> Manual Switch2/1, Multiport Switch/2
  [speedActual] -> MATLAB System2/7
  FromRealSim/3(nVeh) -> [nVehIn]
  [speedActual] -> To Workspace/1, Mux3/2
  [connectionState] -> Display1/1
  Clock/1 -> FromRealSim/1(tSimu), [tSimu]
  [tIn] -> Display3/1
  Bus Selector2/7 -> Scope8/4  "<signalLightDistance>"
  MATLAB System2/4 -> Mux2/2
  Bus Selector2/8 -> Scope8/5  "<signalLightColor>"
  Manual Switch2/1 -> Scope12/1, Multiport Switch/4
  [connectionState] -> MATLAB System2/2, Scope3/1
  MATLAB System2/6 -> Terminator3/1
  Bus Selector2/1 -> MATLAB Function/1(strUint8Vec)  "<linkId>"
  [tIn] -> ToRealSim/1(In1)
  MATLAB System2/2 -> [accelerationCmd], Mux/2  "accelerationDesired"
  MATLAB Function2/1(signalLightIdString) -> Display9/1
  Bus Selector2/2 -> MATLAB Function/2(strLen)  "<linkIdLength>"
  [tIn] -> MATLAB System2/4
  [speedCmd] -> Mux3/3
  Constant4/1 -> Multiport Switch/1
  Manual Switch1/1 -> Mux/1, [speedCmd]
  ToRealSim/2(nMsgSend) -> [nMsgSizeOut]
  FromRealSim/1(simState) -> Display4/1, [simStateIn]
  [speedActual] -> ToRealSim/3(speedDesired)
  FromRealSim/2(t) -> [tIn]
  FromRealSim/5(isVehicleInNetwork) -> [isVehicleInNetwork]
  [accelerationCmd] -> Scope/2
  [VehDataBusIn] -> ToRealSim/2(In2)
  Multiport Switch/1 -> [speedActual]  "speedActual"
  Bus Selector2/6 -> Scope8/3  "<signalLightHeadId>"
  [accelerationActual] -> ToRealSim/4(accelerationDesired)
  ToRealSim/1(ByteSend) -> [ByteDataOut]
  MATLAB Function1/1(intVal) -> Scope8/2
  Bus Selector2/3 -> Scope8/1  "<heading>"
  [isVehicleInNetwork] -> MATLAB System2/6
  Mux3/1 -> Scope/1
  [simStateIn] -> Display2/1
  ? -> MATLAB Function2/2(signalLightIdLength)
  Constant2/1 -> ?
  Manual Switch4/1 -> Manual Switch/2
  [speedDesiredIn] -> Manual Switch/1
  Constant1/1 -> SwitchVehicleSpeed/2(initialSpeed)
  SwitchVehicleSpeed/1(speedCmd) -> Scope4/1, speedCmd/1
  Manual Switch/1 -> SwitchVehicleSpeed/1(speedIn)
  Bus Selector3/1 -> [accelerationDesiredIn]  "<accelerationDesired>"
  Constant3/1 -> Multiport Switch1/1
  [accelerationDesiredIn] -> Multiport Switch1/3
  accelerationActual/1 -> Multiport Switch1/2
  Multiport Switch1/1 -> Scope1/1, [accelerationActual]  "accelerationActual"
  FromRealSim/6(connectionState) -> [connectionState]
  Mux/1 -> Scope2/1
  speedActual/1 -> Manual Switch2/2
  [speedCmd] -> Transfer Fcn/1
  Transfer Fcn/1 -> Multiport Switch/5
  [tSimu] -> MATLAB Function4/4(simulationTime)
  [connectionState] -> MATLAB Function4/3(connectionState), MATLAB Function3/2(connectionState)
  [simStateIn] -> MATLAB Function4/1("simState "), MATLAB Function3/1(simState)
  MATLAB Function3/1(timeStepSimulator) -> Mux1/1, Memory/1
  Memory/1 -> MATLAB Function3/4(timeStepSimulatorPrevious)
  Mux1/1 -> Scope6/1
  MATLAB Function3/2(timeStepTrigger) -> Mux1/2
  Memory1/1 -> MATLAB Function4/2(simStatePrevious)
  MATLAB Function4/2(simState) -> Memory1/1
  [tIn] -> Manual Switch3/2
  Manual Switch3/1 -> Scope9/1, MATLAB Function3/3(timeSimulator)
  [speedCmd] -> Manual Switch4/2

== system CAVE_MachE_dSPACE_250912/TCP SCALEXIO ==
  note: Receiving gas, brake, steering; or three identical speeds
  note: Sending out x, y, heading, time, and speed
  VehOutput : Inport
  comm : Inport  Port=2
  Constant2 : Constant  Value=zeros(1004,1);  OutDataTypeStr=uint8
  Data Type Conversion1 : DataTypeConversion  OutDataTypeStr=double  SaturateOnIntegerOverflow=off  RndMeth=Floor
  Data Type Conversion2 : DataTypeConversion  SaturateOnIntegerOverflow=off  RndMeth=Floor
  Data Type Conversion3 : DataTypeConversion  OutDataTypeStr=boolean  SaturateOnIntegerOverflow=off  RndMeth=Floor
  Defloater{,1..4} (5 alike) : VSIGenLib/Defloater  SystemSampleTime=-1  VariantActivationTime=update diagram  AllowFlexibleInterface=on  Latency=0  AutoFrameSizeCalculation=off
  Demux{,2..5} (5 alike) : Demux
  Demux1 : Demux  Outputs=5
  Display3 : Display
  Ethernet Setup Carla : dsmpblib/Data Inport  Priority=10000
      settings: SourceProductName=dSPACE Model Interface Package for Simulink (MIPS)
  Floater : VSIGenLib/Floater  SystemSampleTime=-1  VariantActivationTime=update diagram  AllowFlexibleInterface=on  Latency=0  AutoFrameSizeCalculation=off
  Floater1 : VSIGenLib/Floater  SystemSampleTime=-1  VariantActivationTime=update diagram  AllowFlexibleInterface=on  Latency=0  AutoFrameSizeCalculation=off
  Floater2 : VSIGenLib/Floater  SystemSampleTime=-1  VariantActivationTime=update diagram  AllowFlexibleInterface=on  Latency=0  AutoFrameSizeCalculation=off
  Mux : Mux  Inputs=21
  Mux1 : Mux  Inputs=3
  Receive [TCP Carla] : dsmpblib/Data Inport  Priority=10000
      settings: SourceProductName=dSPACE Model Interface Package for Simulink (MIPS)
  Scope1 : Scope
  Scope4 : Scope
  Selector1 : Selector  InputPortWidth=1024  IndexOptions=Index vector (dialog)  Indices=[8 7 6 5]  OutputSizes=1
  Selector2 : Selector  InputPortWidth=1024  IndexOptions=Index vector (dialog)  Indices=[12 11 10 9]  OutputSizes=1
  Selector4 : Selector  InputPortWidth=1024  IndexOptions=Index vector (dialog)  Indices=[4 3 2 1]  OutputSizes=1
  SpdAdjust : Gain  Gain=1.1414
  Status/Control_In [TCP Carla] : dsmpblib/Data Inport  Priority=10000
      settings: SourceProductName=dSPACE Model Interface Package for Simulink (MIPS)
  Status/Control_Out [TCP Carla] : dsmpblib/Data Outport  Priority=-10000
      settings: SourceProductName=dSPACE Model Interface Package for Simulink (MIPS)
  Terminator{1..5} (5 alike) : Terminator
  Transmit_In [TCP Carla] : dsmpblib/Data Inport  Priority=10000
      settings: SourceProductName=dSPACE Model Interface Package for Simulink (MIPS)
  Transmit_Out [TCP Carla] : dsmpblib/Data Outport  Priority=-10000
      settings: SourceProductName=dSPACE Model Interface Package for Simulink (MIPS)
  uint8 (unsigned 8) 4 : etargetslib/Byte Pack  datatypes={'uint8'}  byteAlign=1
  Output : Outport
  wires:
  Demux4/4 -> Mux/16
  Demux3/4 -> Mux/12
  Defloater1/1 -> Demux2/1
  Mux/1 -> Data Type Conversion2/1
  Demux4/2 -> Mux/14
  Demux3/1 -> Mux/9
  Demux/4 -> Mux/4
  Demux/1 -> Mux/1
  Demux2/4 -> Mux/8
  Demux1/3 -> Defloater2/1
  Defloater/1 -> Demux/1
  Defloater3/1 -> Demux4/1
  Demux3/3 -> Mux/11
  Demux1/2 -> Defloater1/1
  Demux2/2 -> Mux/6
  Constant2/1 -> uint8 (unsigned 8) 4/1
  Demux1/1 -> Defloater/1
  Defloater2/1 -> Demux3/1
  Demux1/4 -> Defloater3/1
  Demux3/2 -> Mux/10
  Demux/3 -> Mux/3
  Demux/2 -> Mux/2
  VehOutput/1 -> Demux1/1
  Demux2/1 -> Mux/5
  Demux4/1 -> Mux/13
  Demux2/3 -> Mux/7
  Demux4/3 -> Mux/15
  Data Type Conversion2/1 -> Transmit_Out [TCP Carla]/1
  ? -> Terminator2/1
  Transmit_In [TCP Carla]/1 -> Terminator1/1
  Receive [TCP Carla]/1 -> Selector2/1, Selector1/1, Selector4/1
  Selector4/1 -> Floater/1
  Floater/1 -> Display3/1, Mux1/1
  ? -> Terminator4/1
  Data Type Conversion3/1 -> Status/Control_Out [TCP Carla]/1
  comm/1 -> Data Type Conversion3/1
  ? -> Terminator5/1
  ? -> Terminator3/1
  Status/Control_In [TCP Carla]/1 -> Scope4/1
  Ethernet Setup Carla/1 -> Scope1/1
  Demux1/5 -> SpdAdjust/1
  Defloater4/1 -> Demux5/1
  Demux5/2 -> Mux/18
  Demux5/3 -> Mux/19
  Demux5/4 -> Mux/20
  uint8 (unsigned 8) 4/1 -> Mux/21
  Demux5/1 -> Mux/17
  SpdAdjust/1 -> Defloater4/1
  Selector1/1 -> Floater1/1
  Mux1/1 -> Data Type Conversion1/1
  Floater1/1 -> Mux1/2
  Selector2/1 -> Floater2/1
  Floater2/1 -> Mux1/3
  Data Type Conversion1/1 -> Output/1
